simulink model "openManipulatorTorqueCtrlTask"  (R2018a)
settings: Solver=VariableStepAuto  StartTime=0.0  StopTime=20  RelTol=1e-3
PreLoadFcn:
  | openManipulatorParameters;
undefined symbols (not defined in the file): TsCtrl
libraries: OpenManipulatorLib x3, sm_lib x2, nesl_utility x1
settings Model: Creator=scastro  LastModifiedBy=scastro
settings SolverCC: DecoupledContinuousIntegration=on  MinimalZcImpactIntegration=on
settings ExplorerConfigSet: InternalSimMechanicsExplorerSettings="<ExplorerConfiguration><canonicalview>default</canonicalview><AnimationSetting><BasePlaybackSpeed>1.0</BasePlaybackSpeed><PlaybackSpeedFactor>1.0</PlaybackSpeedFactor></AnimationSetting><TilePanel><TileInfo><Tiles Columns=\"1\" Count=\"1\" Rows=\"1\"><Column Weight=\"1\"/><Row Weight=\"1\"/><Tile Height=\"1\" Width=\"1\" X=\"0\" Y=\"0\"/></Tiles></TileInfo><SceneInfo><SceneViewer><BGColor><R>0.60000002384185791</R><G>0.60000002384185791</G><B>0.60000002384185791</B></BGColor><Camera><DoPerspective>off</DoPerspective><Position><X>0.428752942017998073</X><Y>-0.712150369953937545</Y><Z>0.628314823463847372</Z></Position><Center><X>0.0455703138120887447</X><Y>0.0802507835591396851</Y><Z>0.153687090021758288</Z></Center><Up><X>-0.128866037345358619</X><Y>0.462960972240881619</Y><Z>0.876961049648547597</Z></Up><ViewLimDist>1</ViewLimDist><YLim>0.579070269035580121</YLim><XLim>0.64437894599448009</XLim></Camera></SceneViewer></SceneInfo></TilePanel><MechEditorPanel><Cameras/><GfxPanelCameraMap/><VideoCreator><PlaybackSpeedRatio>1.0</PlaybackSpeedRatio><FrameRate>30</FrameRate><VideoFormat>Motion JPEG AVI</VideoFormat><FrameSize>auto</FrameSize></VideoCreator></MechEditorPanel></ExplorerConfiguration>"

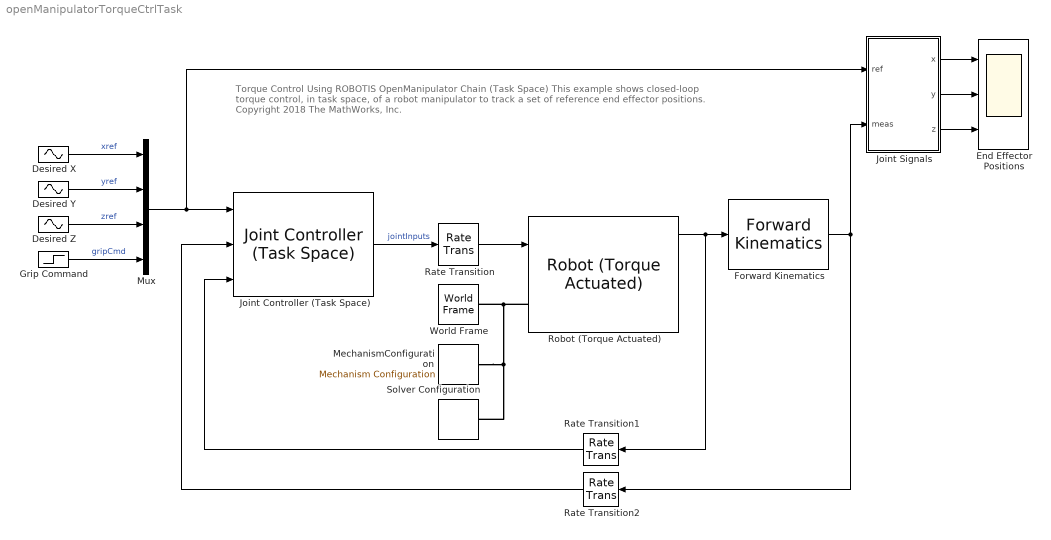
== system openManipulatorTorqueCtrlTask ==
  note: Torque Control Using ROBOTIS OpenManipulator Chain (Task Space)
      |
      | This example shows closed-loop torque control, in task space, of a robot manipulator to track a set of reference end effector positions.
      |
      | Copyright 2018 The MathWorks, Inc.
  Desired X : Sin  Amplitude=0.1  Bias=0.2  Frequency=0.3  Phase=pi/4  SampleTime=TsCtrl
  Desired Y : Sin  Amplitude=0.1  Frequency=0.4  SampleTime=TsCtrl
  Desired Z : Sin  Amplitude=0.05  Bias=0.2  Frequency=0.5  SampleTime=TsCtrl
  End Effector Positions : Scope  NumInputPorts=3
  Forward Kinematics : OpenManipulatorLib/Forward Kinematics
  Grip Command : Step  Time=10  SampleTime=TsCtrl
  Joint Controller (Task Space) : OpenManipulatorLib/Joint Controller (Task Space)  SystemSampleTime=-1  VariantControl=ctrlType==1
  Joint Signals : Subsystem
  MechanismConfiguration : sm_lib/Utilities/Mechanism Configuration  UniformGravity=Constant  GravityVector=[0 0 -9.80665]  GravityUnits=m/s^2  LinearizationDelta=0.001
  Mux : Mux
  Rate Transition : RateTransition
  Rate Transition1 : RateTransition
  Rate Transition2 : RateTransition
  Robot (Torque Actuated) : OpenManipulatorLib/Robot  (Torque Actuated)  SystemSampleTime=-1
  Solver Configuration : nesl_utility/Solver Configuration  PhysicalDomain=network_engine_domain  SubClassName=solver  LeftPortType=input  RightPortType=generic  Tones=[]  Harmonics=[]  SimulateNoise=off  Profile=off  UseLocalSampling=off  EnableSwitchedLinearOptims=on  FrequencyDomain=off  UseCCode=off  RelTol=0.001  AbsTol=1e-06  MinStep=1e-09  ToWorkspace=off  RevertToSquareIcSolve=off  NumHomotopyIterations=100  PhasorMode=off  PhasorModeNumHarmonics=1  DoDC=off  ResidualTolerance=1e-09  UseLocalSolver=off  LocalSolverChoice=NE_BACKWARD_EULER_ADVANCER  LocalSolverSampleTime=0.001  DoFixedCost=off  MaxNonlinIter=3  MaxModeIter=2  LinearAlgebra=Sparse  EquationFormulation=NE_TIME_EF  DelaysMemoryBudget=1024  AutomaticFiltering=on  FilteringTimeConstant=0.001
  World Frame : sm_lib/Frames and Transforms/World Frame
  wires:
  Robot (Torque Actuated)/1 -> Rate Transition1/1, Forward Kinematics/1
  Desired Y/1 -> Mux/2  "yref"
  Desired X/1 -> Mux/1  "xref"
  Rate Transition/1 -> Robot (Torque Actuated)/1
  Mux/1 -> Joint Controller (Task Space)/1, Joint Signals/1(ref)
  Joint Signals/1(x) -> End Effector Positions/1
  Joint Signals/2(y) -> End Effector Positions/2
  Joint Signals/3(z) -> End Effector Positions/3
  Grip Command/1 -> Mux/4  "gripCmd"
  Joint Controller (Task Space)/1 -> Rate Transition/1  "jointInputs"
  Forward Kinematics/1 -> Rate Transition2/1, Joint Signals/2(meas)
  Desired Z/1 -> Mux/3  "zref"
  Rate Transition1/1 -> Joint Controller (Task Space)/3
  Rate Transition2/1 -> Joint Controller (Task Space)/2
  connections:
  Robot (Torque Actuated)/LConn1 -- Solver Configuration/RConn1 -- MechanismConfiguration/RConn1 -- World Frame/RConn1

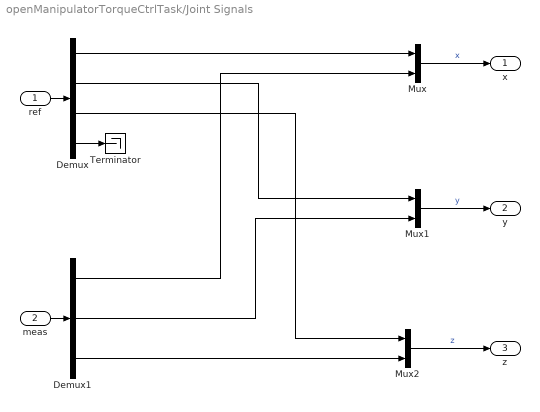
== system openManipulatorTorqueCtrlTask/Joint Signals ==
  ref : Inport
  meas : Inport  Port=2
  Demux : Demux
  Demux1 : Demux  Outputs=3
  Mux : Mux  Inputs=2
  Mux1 : Mux  Inputs=2
  Mux2 : Mux  Inputs=2
  Terminator : Terminator
  x : Outport
  y : Outport  Port=2
  z : Outport  Port=3
  wires:
  Mux2/1 -> z/1  "z"
  ref/1 -> Demux/1
  Mux/1 -> x/1  "x"
  meas/1 -> Demux1/1
  Demux/1 -> Mux/1
  Demux1/1 -> Mux/2
  Mux1/1 -> y/1  "y"
  Demux/2 -> Mux1/1
  Demux1/2 -> Mux1/2
  Demux/3 -> Mux2/1
  Demux1/3 -> Mux2/2
  Demux/4 -> Terminator/1
